simulink subsystem "wheelSlip"  (R2022b)
settings: Solver=VariableStepAuto  StartTime=0.0  StopTime=10.0  RelTol=1e-3
libraries: wheelSpeed_lib x3, Raptor_lib x3
settings Model: Creator=serga  LastModifiedBy=serga

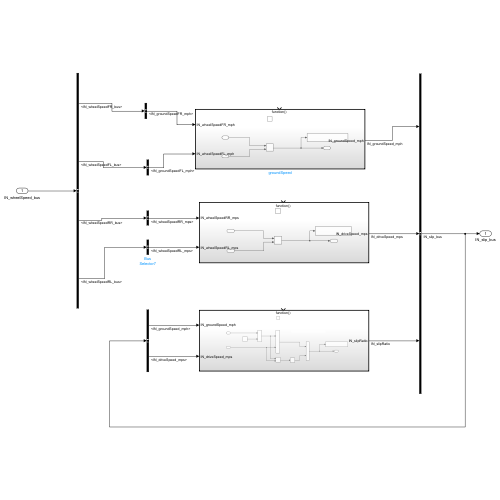
[thumbnail: Simulink's stored preview of the top-level diagram]
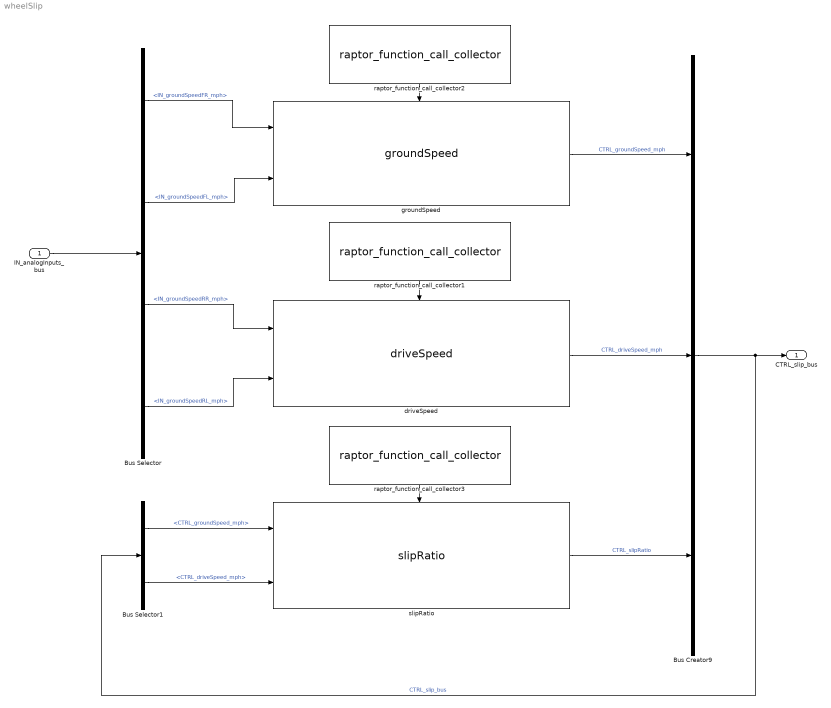
== system wheelSlip ==
  IN_analogInputs_bus : Inport
  Bus Creator9 : BusCreator  Inputs=3
  Bus Selector : BusSelector  OutputSignals=IN_wheelSpeed_bus.IN_wheelSpeedFR_bus.IN_groundSpeedFR_mph,IN_wheelSpeed_bus.IN_wheelSpeedFL_bus.IN_groundSpeedFL_mph,IN_wheelSpeed_bus.IN_wheelSpeedRR_bus.IN_groundSpeedRR_mph,IN_wheelSpeed_bus.IN_wheelSpeedRL_bus.IN_groundSpeedRL_mph
  Bus Selector1 : BusSelector  OutputSignals=CTRL_groundSpeed_mph,CTRL_driveSpeed_mph
  driveSpeed : wheelSpeed_lib/driveSpeed  SystemSampleTime=-1  VariantActivationTime=update diagram  Latency=0  AutoFrameSizeCalculation=off
  groundSpeed : wheelSpeed_lib/groundSpeed  SystemSampleTime=-1  VariantActivationTime=update diagram  Latency=0  AutoFrameSizeCalculation=off
  raptor_function_call_collector1 : Raptor_lib/Triggers/raptor_function_call_collector  count=5
      settings: SourceProductName=Raptor
  raptor_function_call_collector2 : Raptor_lib/Triggers/raptor_function_call_collector  count=5
      settings: SourceProductName=Raptor
  raptor_function_call_collector3 : Raptor_lib/Triggers/raptor_function_call_collector  count=5
      settings: SourceProductName=Raptor
  slipRatio : wheelSpeed_lib/slipRatio  SystemSampleTime=-1  VariantActivationTime=update diagram  Latency=0  AutoFrameSizeCalculation=off
  CTRL_slip_bus : Outport
  wires:
  raptor_function_call_collector3/1 -> slipRatio/Trigger
  raptor_function_call_collector1/1 -> driveSpeed/Trigger
  raptor_function_call_collector2/1 -> groundSpeed/Trigger
  Bus Selector1/1 -> slipRatio/1  "<CTRL_groundSpeed_mph>"
  slipRatio/1 -> Bus Creator9/3  "CTRL_slipRatio"
  Bus Selector1/2 -> slipRatio/2  "<CTRL_driveSpeed_mph>"
  groundSpeed/1 -> Bus Creator9/1  "CTRL_groundSpeed_mph"
  Bus Creator9/1 -> CTRL_slip_bus/1, Bus Selector1/1  "CTRL_slip_bus"
  Bus Selector/2 -> groundSpeed/2  "<IN_groundSpeedFL_mph>"
  IN_analogInputs_bus/1 -> Bus Selector/1
  Bus Selector/1 -> groundSpeed/1  "<IN_groundSpeedFR_mph>"
  driveSpeed/1 -> Bus Creator9/2  "CTRL_driveSpeed_mph"
  Bus Selector/4 -> driveSpeed/2  "<IN_groundSpeedRL_mph>"
  Bus Selector/3 -> driveSpeed/1  "<IN_groundSpeedRR_mph>"
